simulink model "Two_String_Model"  (R2023b)
settings: Solver=VariableStepAuto  StartTime=0.0  StopTime=10.0  RelTol=1e-3
values from neighbouring files (symbols this model uses):
  period_sequence = normalised_period(f_s,zelda)    [main.m]
  T_s = 1/f_s    (= 6.25e-05)    [main.m]
undefined symbols (not defined in the file or in its folder): frac_delay_inter, gaussian
libraries: simulink x3, dspvision x1
settings Model: Creator=andre  LastModifiedBy=andre

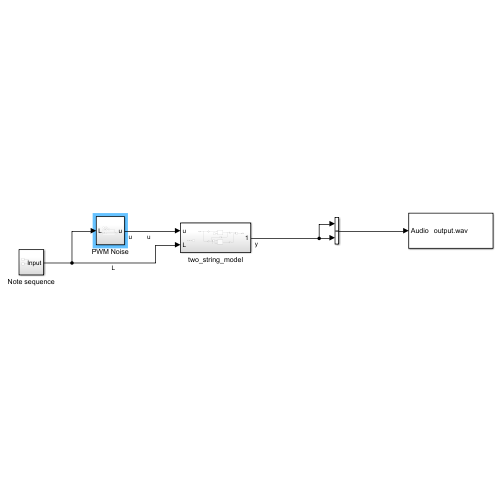
[thumbnail: Simulink's stored preview of the top-level diagram]
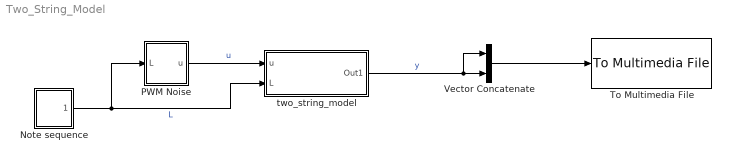
== system Two_String_Model ==
  Note sequence : Subsystem
  PWM Noise : Subsystem
  To Multimedia File : dspvision/To Multimedia File  outputFilename=output.wav  streamSelection=Audio only  videoCompressor=None (uncompressed)  audioCompressor=None (uncompressed)  imagePorts=Separate color signals  fileType=WAV  audioDatatype=16-bit integer  fourcc=RGB  videoQuality=75  mj2000CompFactor=10
      settings: LibrarySourceBlock=dspsnks4/To Multimedia File
  Vector Concatenate : Concatenate
  two_string_model : Subsystem
  wires:
  Note sequence/1(Input) -> two_string_model/2(L), PWM Noise/1(L)  "L"
  PWM Noise/1(u) -> two_string_model/1(u)  "u"
  two_string_model/1(Out1) -> Vector Concatenate/1, Vector Concatenate/2  "y"
  Vector Concatenate/1 -> To Multimedia File/1

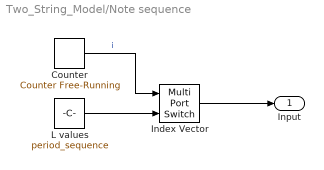
== system Two_String_Model/Note sequence ==
  Counter : simulink/Sources/Counter Free-Running  NumBits=4  tsamp=0.2
  Index Vector : MultiPortSwitch  DataPortOrder=Zero-based contiguous  Inputs=1  zeroidx=on  SaturateOnIntegerOverflow=off  InputSameDT=off
  L values : Constant  Value=period_sequence
  Input : Outport
  wires:
  L values/1 -> Index Vector/2
  Index Vector/1 -> Input/1
  Counter/1 -> Index Vector/1  "i"

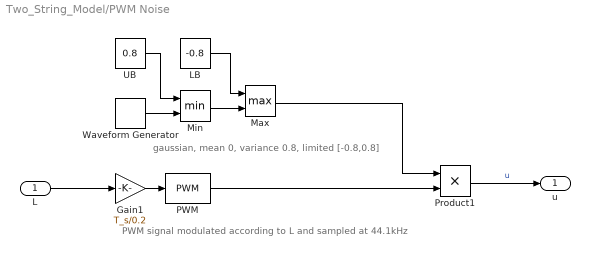
== system Two_String_Model/PWM Noise ==
  note: PWM signal modulated according to L and sampled at 44.1kHz
  note: gaussian, mean 0, variance 0.8, limited [-0.8,0.8]
  L : Inport
  Gain1 : Gain  Gain=T_s/0.2
  LB : Constant  Value=-0.8
  Max : MinMax  Function=max  Inputs=2
  Min : MinMax  Inputs=2
  PWM : simulink/Discontinuities/PWM  DisableCoverage=on  Period=0.2  InitialDelay=0  DisallowZeroDutyCycle=off  RunAtFixedTimeIntervals=on  SampleTime=T_s
  Product1 : Product
  UB : Constant  Value=0.8
  Waveform Generator : simulink/Sources/Waveform Generator  OutMin=[]  OutMax=[]  OutDataTypeStr=double  SelectedSignal=1  Signals=gaussian('Mean',0,'Variance',0.8,'Seed',1)  BlockNames=MultiportSwitch_c96a69a61ea7450  SampleTime=T_s
  u : Outport
  wires:
  LB/1 -> Max/1
  Waveform Generator/1 -> Min/2
  UB/1 -> Min/1
  Min/1 -> Max/2
  PWM/1 -> Product1/2
  Gain1/1 -> PWM/1
  L/1 -> Gain1/1
  Product1/1 -> u/1  "u"
  Max/1 -> Product1/1

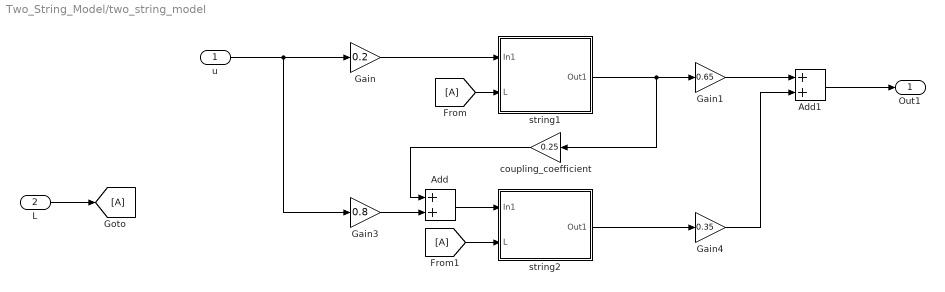
== system Two_String_Model/two_string_model ==
  u : Inport
  L : Inport  Port=2
  Add : Sum
  Add1 : Sum
  From : From
  From1 : From
  Gain : Gain  Gain=0.2
  Gain1 : Gain  Gain=0.65
  Gain3 : Gain  Gain=0.8
  Gain4 : Gain  Gain=0.35
  Goto : Goto
  coupling_coefficient : Gain  Gain=0.25
  string1 : Subsystem
  string2 : Subsystem
  Out1 : Outport
  wires:
  string1/1(Out1) -> coupling_coefficient/1, Gain1/1
  Add/1 -> string2/1(In1)
  u/1 -> Gain/1, Gain3/1
  Gain/1 -> string1/1(In1)
  coupling_coefficient/1 -> Add/1
  Gain3/1 -> Add/2
  string2/1(Out1) -> Gain4/1
  Gain1/1 -> Add1/1
  Add1/1 -> Out1/1
  L/1 -> Goto/1
  From/1 -> string1/2(L)
  From1/1 -> string2/2(L)
  Gain4/1 -> Add1/2

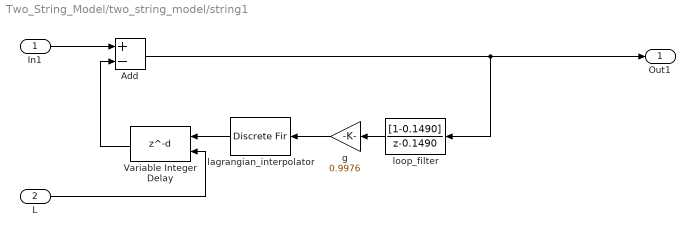
== system Two_String_Model/two_string_model/string1 ==
  In1 : Inport
  L : Inport  Port=2
  Add : Sum  Inputs=+-
  Variable Integer Delay : Delay  DelayLengthSource=Input port  DelayLengthUpperLimit=256  PreventDirectFeedthrough=on  UseCircularBuffer=on
      settings: InputPortMap=u0,p1
  g : Gain  Gain=0.9976
  lagrangian_interpolator : DiscreteFir  Coefficients=frac_delay_inter
  loop_filter : DiscreteTransferFcn  Numerator=[1-0.1490]  Denominator=[1 -0.1490]
  Out1 : Outport
  wires:
  g/1 -> lagrangian_interpolator/1
  Add/1 -> Out1/1, loop_filter/1
  loop_filter/1 -> g/1
  lagrangian_interpolator/1 -> Variable Integer Delay/1
  Variable Integer Delay/1 -> Add/2
  In1/1 -> Add/1
  L/1 -> Variable Integer Delay/2

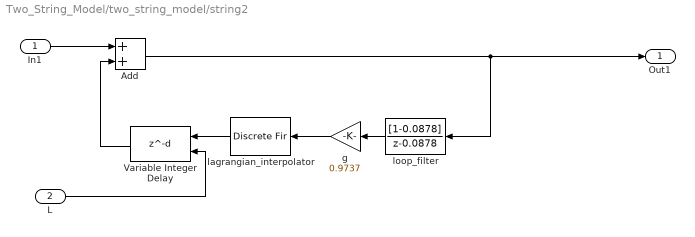
== system Two_String_Model/two_string_model/string2 ==
  In1 : Inport
  L : Inport  Port=2
  Add : Sum
  Variable Integer Delay : Delay  DelayLengthSource=Input port  DelayLengthUpperLimit=256  PreventDirectFeedthrough=on  UseCircularBuffer=on
      settings: InputPortMap=u0,p1
  g : Gain  Gain=0.9737
  lagrangian_interpolator : DiscreteFir  Coefficients=frac_delay_inter
  loop_filter : DiscreteTransferFcn  Numerator=[1-0.0878]  Denominator=[1 -0.0878]
  Out1 : Outport
  wires:
  g/1 -> lagrangian_interpolator/1
  Add/1 -> Out1/1, loop_filter/1
  loop_filter/1 -> g/1
  lagrangian_interpolator/1 -> Variable Integer Delay/1
  Variable Integer Delay/1 -> Add/2
  In1/1 -> Add/1
  L/1 -> Variable Integer Delay/2
